simulink model "session"  (R2022a)
settings: configuration reference "session_config" (kept outside this file)
undefined symbols (not defined in the file): framePeriod_s
settings Model: Creator=remoteuser  LastModifiedBy=remoteuser
settings ConfigSetRef: SourceName=session_config  SourceLocation=Base Workspace

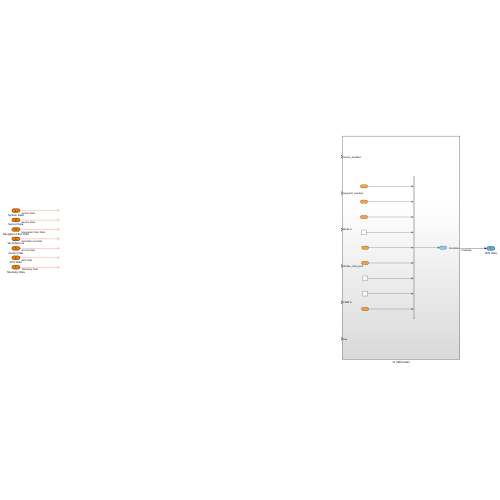
[thumbnail: Simulink's stored preview of the top-level diagram]
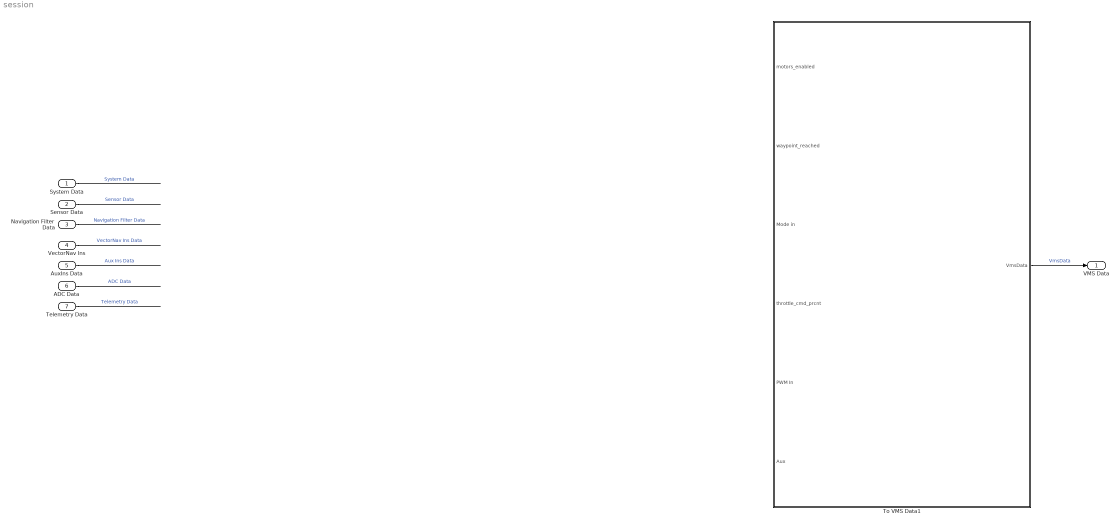
== system session ==
  System Data : Inport  OutDataTypeStr=Bus: SysData  SampleTime=framePeriod_s  BusOutputAsStruct=on
  Sensor Data : Inport  Port=2  OutDataTypeStr=Bus: SensorData  SampleTime=framePeriod_s  BusOutputAsStruct=on
  Navigation Filter Data : Inport  Port=3  OutDataTypeStr=Bus: InsData  SampleTime=framePeriod_s  BusOutputAsStruct=on
  VectorNav Ins : Inport  Port=4  OutDataTypeStr=Bus: InsData  SampleTime=framePeriod_s  BusOutputAsStruct=on
  AuxIns Data : Inport  Port=5  OutDataTypeStr=Bus: AuxInsData  SampleTime=framePeriod_s  BusOutputAsStruct=on
  ADC Data : Inport  Port=6  OutDataTypeStr=Bus: AdcData  SampleTime=framePeriod_s  BusOutputAsStruct=on
  Telemetry Data : Inport  Port=7  OutDataTypeStr=Bus: TelemData  SampleTime=framePeriod_s  BusOutputAsStruct=on
  To VMS Data1 : Subsystem
  VMS Data : Outport  OutDataTypeStr=Bus: VmsData  SampleTime=framePeriod_s  BusOutputAsStruct=on
  wires:
  System Data/1 -> ?  "System Data"
  Navigation Filter Data/1 -> ?  "Navigation Filter Data"
  ADC Data/1 -> ?  "ADC Data"
  Sensor Data/1 -> ?  "Sensor Data"
  VectorNav Ins/1 -> ?  "VectorNav Ins Data"
  AuxIns Data/1 -> ?  "Aux Ins Data"
  Telemetry Data/1 -> ?  "Telemetry Data"
  To VMS Data1/1(VmsData) -> VMS Data/1  "VmsData"

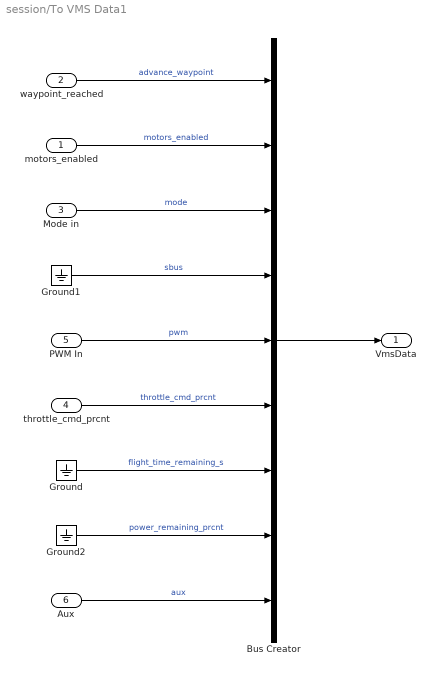
== system session/To VMS Data1 ==
  motors_enabled : Inport
  waypoint_reached : Inport  Port=2
  Mode in : Inport  Port=3
  throttle_cmd_prcnt : Inport  Port=4
  PWM In : Inport  Port=5
  Aux : Inport  Port=6
  Bus Creator : BusCreator  Inputs=9  OutDataTypeStr=Bus: VmsData  NonVirtualBus=on
      settings: InheritFromInputs=off
  Ground : Ground
  Ground1 : Ground
  Ground2 : Ground
  VmsData : Outport
  wires:
  Bus Creator/1 -> VmsData/1
  waypoint_reached/1 -> Bus Creator/1  "advance_waypoint"
  motors_enabled/1 -> Bus Creator/2  "motors_enabled"
  Mode in/1 -> Bus Creator/3  "mode"
  Ground1/1 -> Bus Creator/4  "sbus"
  PWM In/1 -> Bus Creator/5  "pwm"
  throttle_cmd_prcnt/1 -> Bus Creator/6  "throttle_cmd_prcnt"
  Aux/1 -> Bus Creator/9  "aux"
  Ground/1 -> Bus Creator/7  "flight_time_remaining_s"
  Ground2/1 -> Bus Creator/8  "power_remaining_prcnt"
